simulink model "cp_wideband_gammatone_filter"  (R2020b)
settings: Solver=FixedStepDiscrete  StartTime=0.0  StopTime=stopTime  FixedStep=2.0833333333333333e-05  RelTol=1e-3
undefined symbols (not defined in the file or in its folder): cf, cordiciterationswb, delta_phase, jsin, TauWBMax, tdres, wborder
settings Model: Creator=Ross  LastModifiedBy=conno
settings DataIOCC: SaveOutput=off  SaveTime=off  ReturnWorkspaceOutputs=off
settings OptimizationCC: BlockReduction=off  ConditionallyExecuteInputs=off  DefaultParameterBehavior=Inlined
settings DebuggingCC: ReadBeforeWriteMsg=DisableAll  WriteAfterWriteMsg=DisableAll  WriteAfterReadMsg=DisableAll  AlgebraicLoopMsg=error  MultiTaskDSMMsg=none  SingleTaskRateTransMsg=error  PregeneratedLibrarySubsystemCodeDiagnostic=none  ArithmeticOperatorsInVariantConditions=warning
settings HardwareCC: ProdBitPerPointer=32  ProdBitPerSizeT=32  ProdBitPerPtrDiffT=32  ProdLargestAtomicFloat=None  ProdIntDivRoundTo=Undefined  ProdEndianess=Unspecified  ProdWordSize=32  ProdHWDeviceType=ASIC/FPGA->ASIC/FPGA  TargetBitPerPointer=64  TargetBitPerSizeT=64  TargetBitPerPtrDiffT=64  TargetLongLongMode=on  TargetIntDivRoundTo=Zero  TargetEndianess=LittleEndian  TargetWordSize=64  TargetHWDeviceType=Custom Processor->MATLAB Host Computer  ProdEqTarget=off
settings ModelReferenceCC: UpdateModelReferenceTargets=IfOutOfDate
settings SFSimCC: SFSimEcho=off  SimUseLocalCustomCode=off  CustomCodeUndefinedFunction=UseInterfaceOnly
settings RTWCC: RTWUseLocalCustomCode=off

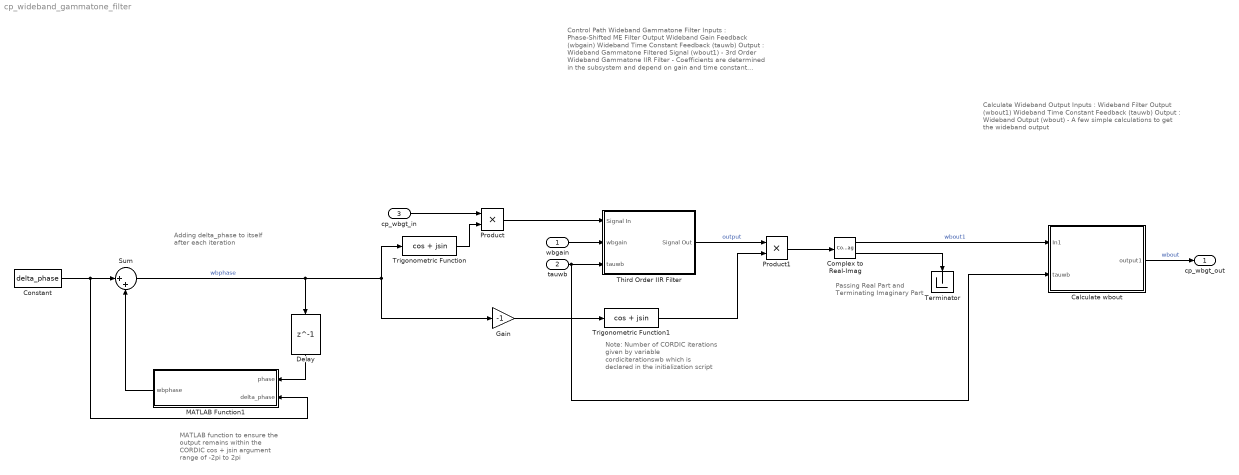
== system cp_wideband_gammatone_filter ==
  note: Calculate Wideband Output
      |
      | Inputs : Wideband Filter Output (wbout1)
      | Wideband Time Constant Feedback (tauwb)
      |
      | Output : Wideband Output (wbout)
      |
      | - A few simple calculations to get the wideband output
  note: Control Path Wideband Gammatone Filter
      |
      | Inputs : Phase-Shifted ME Filter Output
      | Wideband Gain Feedback (wbgain)
      | Wideband Time Constant Feedback (tauwb)
      |
      | Output : Wideband Gammatone Filtered Signal (wbout1)
      |
      | - 3rd Order Wideband Gammatone IIR Filter
      |
      | - Coefficients are determined in the subsystem and depend on gain and time constant feedback
      |
      | - Implemented w/ Direct Form I Block Structure
  note: MATLAB function to ensure the output remains within the CORDIC cos + jsin argument range of -2pi to 2pi
  note: Adding delta_phase to itself after each iteration
  note: Note: Number of CORDIC iterations given by variable cordiciterationswb which is declared in the initialization script
  note: Passing Real Part and Terminating Imaginary Part
  wbgain : Inport  OutDataTypeStr=single  PortDimensions=1  SampleTime=[2.0833333333333333e-05,0]
  tauwb : Inport  Port=2  OutDataTypeStr=single  PortDimensions=1  SampleTime=[2.0833333333333333e-05,0]
  cp_wbgt_in : Inport  Port=3  OutDataTypeStr=single  PortDimensions=1  SampleTime=[2.0833333333333333e-05,0]
  Calculate wbout : Subsystem
  Complex to Real-Imag : ComplexToRealImag
  Constant : Constant  Value=delta_phase  OutDataTypeStr=single  SampleTime=-1
  Delay : Delay  DelayLength=1  InitialCondition=0  UseCircularBuffer=on
  Gain : Gain  Gain=-1  OutDataTypeStr=single
  MATLAB Function1 : MATLAB Function  TreatAsAtomicUnit=on
  Product : Product  OutDataTypeStr=single
  Product1 : Product  OutDataTypeStr=single
  Sum : Sum  Inputs=|++  OutDataTypeStr=single
  Terminator : Terminator
  Third Order IIR Filter : Subsystem
  Trigonometric Function : Trigonometry  Operator=cos + jsin  NumberOfIterations=cordiciterationswb
  Trigonometric Function1 : Trigonometry  Operator=cos + jsin  NumberOfIterations=cordiciterationswb
  cp_wbgt_out : Outport  OutDataTypeStr=single  PortDimensions=1  SampleTime=[2.0833333333333333e-05,0]  VectorParamsAs1DForOutWhenUnconnected=off
  wires:
  MATLAB Function1/1(wbphase) -> Sum/2
  Delay/1 -> MATLAB Function1/1(phase)
  wbgain/1 -> Third Order IIR Filter/2(wbgain)
  tauwb/1 -> Third Order IIR Filter/3(tauwb), Calculate wbout/2(tauwb)
  Trigonometric Function1/1 -> Product1/2
  Gain/1 -> Trigonometric Function1/1
  Complex to Real-Imag/2 -> Terminator/1
  Product1/1 -> Complex to Real-Imag/1
  Sum/1 -> Gain/1, Trigonometric Function/1, Delay/1  "wbphase"
  Product/1 -> Third Order IIR Filter/1(Signal In)
  cp_wbgt_in/1 -> Product/1
  Constant/1 -> Sum/1, MATLAB Function1/2(delta_phase)
  Trigonometric Function/1 -> Product/2
  Third Order IIR Filter/1(Signal Out) -> Product1/1  "output"
  Complex to Real-Imag/1 -> Calculate wbout/1(In1)  "wbout1"
  Calculate wbout/1(output1) -> cp_wbgt_out/1  "wbout"

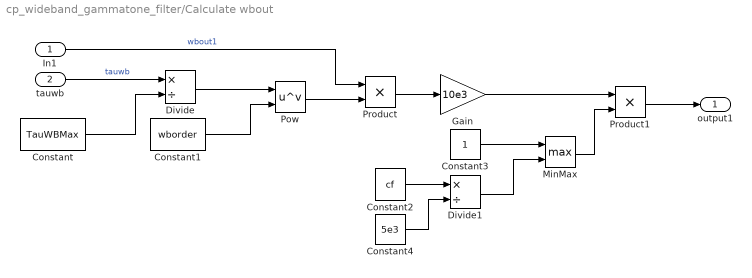
== system cp_wideband_gammatone_filter/Calculate wbout ==
  In1 : Inport
  tauwb : Inport  Port=2
  Constant : Constant  Value=TauWBMax  OutDataTypeStr=single  SampleTime=-1
  Constant1 : Constant  Value=wborder  OutDataTypeStr=single  SampleTime=-1
  Constant2 : Constant  Value=cf  OutDataTypeStr=single  SampleTime=-1
  Constant3 : Constant  OutDataTypeStr=single  SampleTime=-1
  Constant4 : Constant  Value=5e3  OutDataTypeStr=single  SampleTime=-1
  Divide : Product  Inputs=*/  RndMeth=Zero  SaturateOnIntegerOverflow=on
  Divide1 : Product  Inputs=*/  RndMeth=Zero  SaturateOnIntegerOverflow=on
  Gain : Gain  Gain=10e3
  MinMax : MinMax  Function=max  Inputs=2
  Pow : Math  Operator=pow  SignedPower=on  RndMeth=Zero  SaturateOnIntegerOverflow=on
  Product : Product
  Product1 : Product
  output1 : Outport  VectorParamsAs1DForOutWhenUnconnected=off
  wires:
  Constant4/1 -> Divide1/2
  Constant2/1 -> Divide1/1
  Product1/1 -> output1/1
  MinMax/1 -> Product1/2
  Constant3/1 -> MinMax/1
  Divide1/1 -> MinMax/2
  Gain/1 -> Product1/1
  Product/1 -> Gain/1
  Pow/1 -> Product/2
  Constant1/1 -> Pow/2
  Divide/1 -> Pow/1
  Constant/1 -> Divide/2
  In1/1 -> Product/1  "wbout1"
  tauwb/1 -> Divide/1  "tauwb"

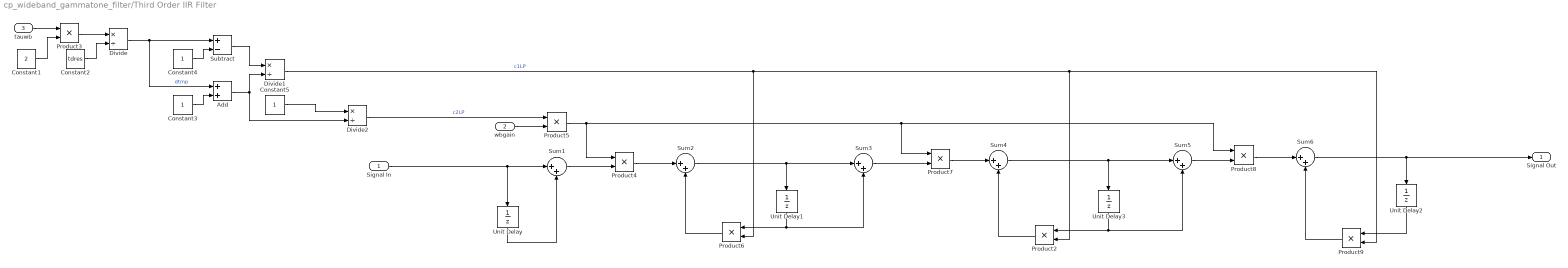
== system cp_wideband_gammatone_filter/Third Order IIR Filter ==
  Signal In : Inport
  wbgain : Inport  Port=2
  tauwb : Inport  Port=3
  Add : Sum
  Constant1 : Constant  Value=2  OutDataTypeStr=single  SampleTime=-1
  Constant2 : Constant  Value=tdres  OutDataTypeStr=single  SampleTime=-1
  Constant3 : Constant  OutDataTypeStr=single  SampleTime=-1
  Constant4 : Constant  OutDataTypeStr=single  SampleTime=-1
  Constant5 : Constant  OutDataTypeStr=single  SampleTime=-1
  Divide : Product  Inputs=*/  RndMeth=Zero  SaturateOnIntegerOverflow=on
  Divide1 : Product  Inputs=*/  RndMeth=Zero  SaturateOnIntegerOverflow=on
  Divide2 : Product  Inputs=*/  RndMeth=Zero  SaturateOnIntegerOverflow=on
  Product{2..9} (8 alike) : Product
  Subtract : Sum  Inputs=+-
  Sum{1..6} (6 alike) : Sum  Inputs=|++
  Unit Delay{,1..3} (4 alike) : UnitDelay  SampleTime=-1  HasFrameUpgradeWarning=on
  Signal Out : Outport  VectorParamsAs1DForOutWhenUnconnected=off
  wires:
  Sum6/1 -> Signal Out/1, Unit Delay2/1
  Product8/1 -> Sum6/1
  Subtract/1 -> Divide1/1
  Product2/1 -> Sum4/2
  Signal In/1 -> Unit Delay/1, Sum1/1
  Product5/1 -> Product4/1, Product7/1, Product8/1
  Constant1/1 -> Product3/2
  Divide2/1 -> Product5/1  "c2LP"
  Unit Delay/1 -> Sum1/2
  Divide/1 -> Add/1, Subtract/1  "dtmp"
  Sum3/1 -> Product7/2
  Add/1 -> Divide2/2, Divide1/2
  Sum5/1 -> Product8/2
  Unit Delay1/1 -> Sum3/2, Product6/1
  Constant5/1 -> Divide2/1
  Product7/1 -> Sum4/1
  Product9/1 -> Sum6/2
  Unit Delay3/1 -> Sum5/2, Product2/1
  Sum2/1 -> Sum3/1, Unit Delay1/1
  Product6/1 -> Sum2/2
  Sum4/1 -> Sum5/1, Unit Delay3/1
  tauwb/1 -> Product3/1
  Product3/1 -> Divide/1
  Constant4/1 -> Subtract/2
  wbgain/1 -> Product5/2
  Unit Delay2/1 -> Product9/1
  Product4/1 -> Sum2/1
  Constant2/1 -> Divide/2
  Sum1/1 -> Product4/2
  Constant3/1 -> Add/2
  Divide1/1 -> Product6/2, Product9/2, Product2/2  "c1LP"

== matlab function cp_wideband_gammatone_filter/MATLAB Function1 ==
  data: phase input; wbphase output; delta_phase input
% Matthew Blunt
% Speech % Hearing Internship
% Check Gammatone Cosine Argument
% 6/6/2019

% ---------------------------------------------------------------------- %
% NOTES: 
% ---------------------------------------------------------------------- %

% The following script is designed to work within the CP Wideband Gammatone
% Filter Simulink model in order to ensure that the argument of the
% trigonometric representation of a complex exponential remains within
% [-2pi,2pi). The function will simply take in the wb phase variable and
% output the same value in radians that falls within the range of arguments
% for the Simulink trigonometric block.

% *** NOTE: Edited by Matthew Blunt 03/05/2020
% *** Now evaluates bounds in the feedback loop to ensure stability for
% FPGA implementation

% ---------------------------------------------------------------------- %
% CODE: 
% ---------------------------------------------------------------------- %

% *** Edited by Matthew Blunt 03/05/2020
% *** Only accounts for negative values of delta_phase
function wbphase = WbGammaToneCosineArgCheck(phase,delta_phase)
    if phase <= (-2*pi - delta_phase)
        phase = phase+2*pi;
    end
    wbphase = phase;
end
